simulink model "new_pll_fs"  (Simulink 7.5)
settings: Solver=ode45  StartTime=0.0  StopTime=inf  RelTol=1e-3
undefined symbols (not defined in the file or in its folder): get
libraries: simulink x6, powerlib_extras x2, commsynccomp2 x2, dspsnks4 x2, dsparch4 x1
CloseFcn:
  | rtwprivate ssgencode ModelCloseRequest new_pll_fs
settings Model: Creator=Administrator  LastModifiedBy=kostas777711  SimulationMode=accelerator
settings OptimizationCC: InitFltsAndDblsToZero=on
settings DebuggingCC: SaveWithParameterizedLinksMsg=none  SolverPrmCheckMsg=none  SigSpecEnsureSampleTimeMsg=none  StrictBusMsg=Warning
settings HardwareCC: ProdIntDivRoundTo=Zero  ProdEndianess=LittleEndian  ProdHWDeviceType=32-bit xPC Target (AMD Athlon)  TargetEndianess=LittleEndian  TargetHWDeviceType=MATLAB Host  ProdEqTarget=off
settings RTWCC: SystemTargetFile=accel.tlc  TemplateMakefile=accel_default_tmf  RTWVerbose=off  ProcessScript=accel_make_rtw_hook
settings STFCustomTargetCC: TargetFcnLib=ansi_tfl_tmw.mat  GeneratePreprocessorConditionals=Disable all  SystemTargetFile=accel.tlc

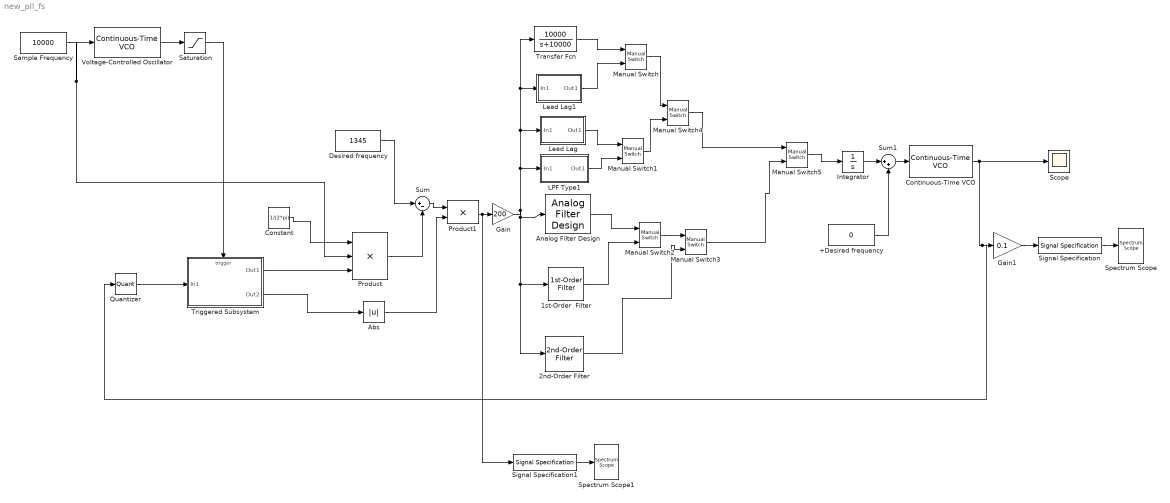
== system new_pll_fs ==
  +Desired frequency : Constant  Value=0  OutDataType=sfix(16)  OutScaling=2^0
  1st-Order  Filter : powerlib_extras/Control  Blocks/1st-Order  Filter  DialogController=POWERSYS.PowerSysDialog  SystemSampleTime=-1  FilterType=Highpass  Tc=12e-3  Initialize=off  Vac_Init=[0.8 -25 60]  Vdc_Init=-0.4  PlotResponse=off  param1=[1 500 1]
  2nd-Order Filter : powerlib_extras/Control  Blocks/2nd-Order Filter  DialogController=POWERSYS.PowerSysDialog  SystemSampleTime=-1  FilterType=Lowpass  Fo=500  Zeta=0.707  Initialize=off  Vac_Init=[1 45 60]  Vdc_Init=-0.5  PlotResponse=off  param1=[1 500 1]
  Abs : Abs  SaturateOnIntegerOverflow=on
  Analog Filter Design : dsparch4/Analog Filter Design  method=Butterworth  filttype=Lowpass  N=4  Wlo=5000  Whi=80  Rp=2  Rs=40
  Constant : Constant  Value=1/(2*pi)  OutDataType=sfix(16)  OutScaling=2^0
  Continuous-Time VCO : commsynccomp2/Continuous-Time VCO  SystemSampleTime=-1  Ac=1  Fc=0  Kc=1  Ph=0
  Desired frequency : Constant  Value=1345  OutDataType=sfix(16)  OutScaling=2^0
  Gain : Gain  Gain=200  ParameterDataType=sfix(16)  ParameterScaling=2^0  OutDataType=sfix(16)  OutScaling=2^0  SaturateOnIntegerOverflow=on  OutDataTypeStr=Inherit: Same as input  ParamDataTypeStr=Inherit: Same as input
  Gain1 : Gain  Gain=0.1  ParameterDataType=sfix(16)  ParameterScaling=2^0  OutDataType=sfix(16)  OutScaling=2^0  SaturateOnIntegerOverflow=on  OutDataTypeStr=Inherit: Same as input  ParamDataTypeStr=Inherit: Same as input
  Integrator : Integrator
  LPF Type1 : Subsystem  TreatAsAtomicUnit=on
  Lead Lag : Subsystem  TreatAsAtomicUnit=on
  Lead Lag1 : Subsystem  TreatAsAtomicUnit=on
  Manual Switch{,2..4} (4 alike) : simulink/Signal Routing/Manual Switch  SystemSampleTime=-1  sw=1  action=0  varsize=off
  Manual Switch1 : simulink/Signal Routing/Manual Switch  SystemSampleTime=-1  sw=0  action=0  varsize=off
  Manual Switch5 : simulink/Signal Routing/Manual Switch  SystemSampleTime=-1  sw=0  action=0  varsize=off
  Product : Product  Inputs=3  OutDataType=sfix(16)  OutScaling=2^0  SaturateOnIntegerOverflow=on  OutDataTypeStr=Inherit: Same as first input
  Product1 : Product  OutDataType=sfix(16)  OutScaling=2^0  SaturateOnIntegerOverflow=on  OutDataTypeStr=Inherit: Same as first input
  Quantizer : Quantizer  QuantizationInterval=2/(2^8)
  Sample Frequency : Constant  Value=10000  OutDataType=sfix(16)  OutScaling=2^0
  Saturation : Saturate  UpperLimit=1  LowerLimit=-1
  Scope : Scope
      settings: TimeRange=0.002973977695167286  YMin=-1  YMax=1
  Signal Specification : SignalSpecification  Dimensions=1  SampleTime=1/10000  OutDataType=sfix(16)  OutScaling=2^0
  Signal Specification1 : SignalSpecification  Dimensions=1  SampleTime=1/10000  OutDataType=sfix(16)  OutScaling=2^0
  Spectrum Scope : dspsnks4/Spectrum Scope  DialogController=dspdialog.SpectrumScope  DialogControllerArgs=DataTag0  SystemSampleTime=-1  ScopeProperties=on  Domain=Frequency  HorizSpan=1  UseBuffer=on  BufferSize=2048  Overlap=64  inpFftLenInherit=on  FFTlength=2048  numAvg=2  DisplayProperties=off  AxisGrid=on  Memory=off  FrameNumber=on  AxisLegend=off  AxisZoom=off  OpenScopeAtSimStart=on  OpenScopeImmediately=off  FigPos=get(0,'defaultfigureposition')  AxisProperties=off  XUnits=Hertz  XRange=[0...Fs/2]  XDisplay=0  InheritXIncr=on  XIncr=1.0  XLabel=Samples  XLimit=Auto  YUnits=dBW/Hertz  XMax=1  XMin=0  YLabel=Magnitude, dB  LineProperties=off  LineColors=[1 0 0]  wintypeSpecScope=Hann  RsSpecScope=50  betaSpecScope=5  winsampSpecScope=Periodic  XAxisParamsVer=6.8
      settings: YMin=-204.6096  YMax=-26.407
  Spectrum Scope1 : dspsnks4/Spectrum Scope  DialogController=dspdialog.SpectrumScope  DialogControllerArgs=DataTag1  SystemSampleTime=-1  ScopeProperties=on  Domain=Frequency  HorizSpan=1  UseBuffer=on  BufferSize=2048  Overlap=64  inpFftLenInherit=on  FFTlength=2048  numAvg=2  DisplayProperties=off  AxisGrid=on  Memory=off  FrameNumber=on  AxisLegend=off  AxisZoom=off  OpenScopeAtSimStart=on  OpenScopeImmediately=off  FigPos=get(0,'defaultfigureposition')  AxisProperties=off  XUnits=Hertz  XRange=[0...Fs/2]  XDisplay=0  InheritXIncr=on  XIncr=1.0  XLabel=Samples  XLimit=Auto  YUnits=dBW/Hertz  XMax=1  XMin=0  YLabel=Magnitude, dB  LineProperties=off  LineStyles=-  LineMarkers=.  wintypeSpecScope=Hann  RsSpecScope=50  betaSpecScope=5  winsampSpecScope=Periodic  XAxisParamsVer=6.8
      settings: YMin=-177.2819  YMax=-38.6723
  Sum : Sum  Inputs=|+-  OutDataType=sfix(16)  OutScaling=2^0  SaturateOnIntegerOverflow=on
  Sum1 : Sum  Inputs=|++  OutDataType=sfix(16)  OutScaling=2^0  SaturateOnIntegerOverflow=on
  Transfer Fcn : TransferFcn  Numerator=[10000]  Denominator=[1 10000]
  Triggered Subsystem : Subsystem  TreatAsAtomicUnit=on
  Voltage-Controlled Oscillator : commsynccomp2/Continuous-Time VCO  SystemSampleTime=-1  Ac=1  Fc=0  Kc=1  Ph=0
  wires:
  Signal Specification/1 -> Spectrum Scope/1
  Gain1/1 -> Signal Specification/1
  Transfer Fcn/1 -> Manual Switch/1
  Lead Lag1/1(Out1) -> Manual Switch/2
  Lead Lag/1(Out1) -> Manual Switch1/1
  LPF Type1/1(Out1) -> Manual Switch1/2
  Analog Filter Design/1 -> Manual Switch2/1
  1st-Order  Filter/1 -> Manual Switch2/2
  Manual Switch2/1 -> Manual Switch3/1
  2nd-Order Filter/1 -> Manual Switch3/2
  Manual Switch/1 -> Manual Switch4/1
  Manual Switch1/1 -> Manual Switch4/2
  Manual Switch4/1 -> Manual Switch5/1
  Continuous-Time VCO/1 -> Scope/1, Gain1/1, Quantizer/1
  Manual Switch3/1 -> Manual Switch5/2
  Signal Specification1/1 -> Spectrum Scope1/1
  Voltage-Controlled Oscillator/1 -> Saturation/1
  Sample Frequency/1 -> Voltage-Controlled Oscillator/1, Product/2
  Desired frequency/1 -> Sum/1
  Product/1 -> Sum/2
  Manual Switch5/1 -> Integrator/1
  Product1/1 -> Gain/1, Signal Specification1/1
  Sum/1 -> Product1/1
  Abs/1 -> Product1/2
  Constant/1 -> Product/1
  Saturation/1 -> Triggered Subsystem/Trigger
  Quantizer/1 -> Triggered Subsystem/1(In1)
  Triggered Subsystem/1(Out1) -> Product/3
  Gain/1 -> Transfer Fcn/1, Lead Lag1/1(In1), Lead Lag/1(In1), LPF Type1/1(In1), Analog Filter Design/1, 1st-Order  Filter/1, 2nd-Order Filter/1
  Triggered Subsystem/2(Out2) -> Abs/1
  Sum1/1 -> Continuous-Time VCO/1
  Integrator/1 -> Sum1/1
  +Desired frequency/1 -> Sum1/2

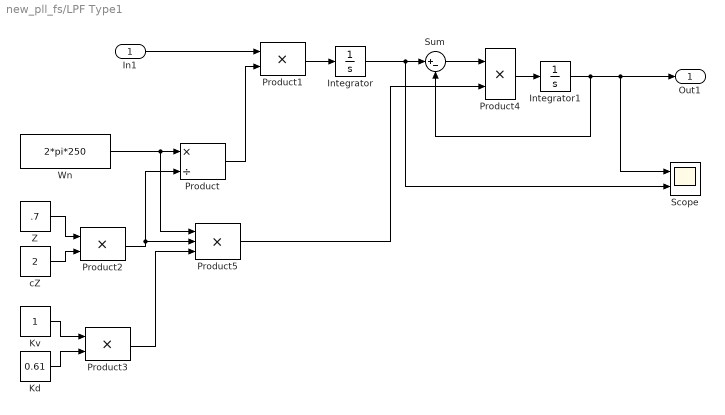
== system new_pll_fs/LPF Type1 ==
  In1 : Inport  OutDataType=sfix(16)  OutScaling=2^0
  Integrator : Integrator  InitialCondition=2500  LimitOutput=on  UpperSaturationLimit=5000  LowerSaturationLimit=10
  Integrator1 : Integrator  InitialCondition=100  LimitOutput=on  UpperSaturationLimit=5000  LowerSaturationLimit=10
  Kd : Constant  Value=0.61  OutDataType=sfix(16)  OutScaling=2^0
  Kv : Constant  OutDataType=sfix(16)  OutScaling=2^0
  Product : Product  Inputs=*/  OutDataType=sfix(16)  OutScaling=2^0  RndMeth=Nearest  SaturateOnIntegerOverflow=on  OutDataTypeStr=Inherit: Same as first input
  Product1 : Product  OutDataType=sfix(16)  OutScaling=2^0  SaturateOnIntegerOverflow=on  OutDataTypeStr=Inherit: Same as first input
  Product2 : Product  OutDataType=sfix(16)  OutScaling=2^0  SaturateOnIntegerOverflow=on  OutDataTypeStr=Inherit: Same as first input
  Product3 : Product  OutDataType=sfix(16)  OutScaling=2^0  SaturateOnIntegerOverflow=on  OutDataTypeStr=Inherit: Same as first input
  Product4 : Product  Inputs=**  OutDataType=sfix(16)  OutScaling=2^0  SaturateOnIntegerOverflow=on  OutDataTypeStr=Inherit: Same as first input
  Product5 : Product  Inputs=***  OutDataType=sfix(16)  OutScaling=2^0  RndMeth=Nearest  SaturateOnIntegerOverflow=on  OutDataTypeStr=Inherit: Same as first input
  Scope : Scope  NumInputPorts=2
      settings: TimeRange=0.01  YMin=748.5~748  YMax=751~753  SaveName=ScopeData2
  Sum : Sum  Inputs=|+-  OutDataType=sfix(16)  OutScaling=2^0  SaturateOnIntegerOverflow=on
  Wn : Constant  Value=2*pi*250  OutDataType=sfix(16)  OutScaling=2^0
  Z : Constant  Value=.7  OutDataType=sfix(16)  OutScaling=2^0
  cZ : Constant  Value=2  OutDataType=sfix(16)  OutScaling=2^0
  Out1 : Outport  OutDataType=sfix(16)  OutScaling=2^0
  wires:
  Product/1 -> Product1/2
  Z/1 -> Product2/1
  cZ/1 -> Product2/2
  Kv/1 -> Product3/1
  Kd/1 -> Product3/2
  Wn/1 -> Product/1, Product5/1
  Product1/1 -> Integrator/1
  Integrator/1 -> Sum/1, Scope/2
  In1/1 -> Product1/1
  Integrator1/1 -> Sum/2, Out1/1, Scope/1
  Sum/1 -> Product4/1
  Product4/1 -> Integrator1/1
  Product2/1 -> Product/2, Product5/2
  Product3/1 -> Product5/3
  Product5/1 -> Product4/2

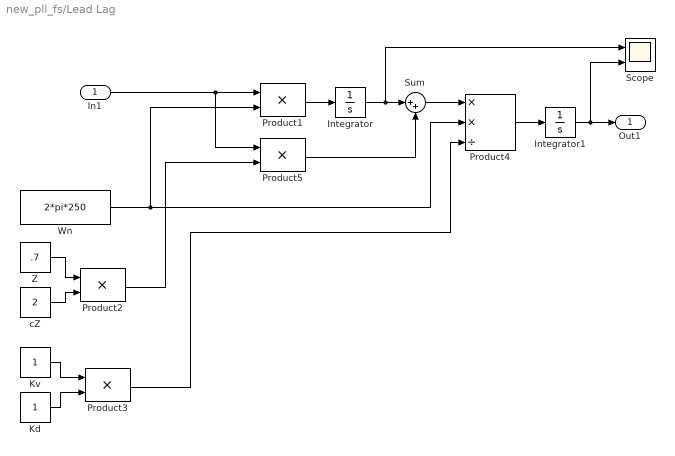
== system new_pll_fs/Lead Lag ==
  In1 : Inport  OutDataType=sfix(16)  OutScaling=2^0
  Integrator : Integrator  UpperSaturationLimit=10  LowerSaturationLimit=-10  ZeroCross=off
  Integrator1 : Integrator  InitialCondition=1000  LimitOutput=on  UpperSaturationLimit=5000  LowerSaturationLimit=10
  Kd : Constant  OutDataType=sfix(16)  OutScaling=2^0
  Kv : Constant  OutDataType=sfix(16)  OutScaling=2^0
  Product{1..3,5} (4 alike) : Product  OutDataType=sfix(16)  OutScaling=2^0  SaturateOnIntegerOverflow=on  OutDataTypeStr=Inherit: Same as first input
  Product4 : Product  Inputs=**/  OutDataType=sfix(16)  OutScaling=2^0  SaturateOnIntegerOverflow=on  OutDataTypeStr=Inherit: Same as first input
  Scope : Scope  NumInputPorts=2
      settings: TimeRange=0.02  YMin=-10~490  YMax=7.5~515  SaveName=ScopeData3
  Sum : Sum  Inputs=|++  OutDataType=sfix(16)  OutScaling=2^0  SaturateOnIntegerOverflow=on
  Wn : Constant  Value=2*pi*250  OutDataType=sfix(16)  OutScaling=2^0
  Z : Constant  Value=.7  OutDataType=sfix(16)  OutScaling=2^0
  cZ : Constant  Value=2  OutDataType=sfix(16)  OutScaling=2^0
  Out1 : Outport  OutDataType=sfix(16)  OutScaling=2^0
  wires:
  Z/1 -> Product2/1
  cZ/1 -> Product2/2
  Kv/1 -> Product3/1
  Kd/1 -> Product3/2
  Wn/1 -> Product1/2, Product4/2
  Product1/1 -> Integrator/1
  In1/1 -> Product1/1, Product5/1
  Integrator/1 -> Sum/1, Scope/1
  Product2/1 -> Product5/2
  Product5/1 -> Sum/2
  Sum/1 -> Product4/1
  Product3/1 -> Product4/3
  Product4/1 -> Integrator1/1
  Integrator1/1 -> Out1/1, Scope/2

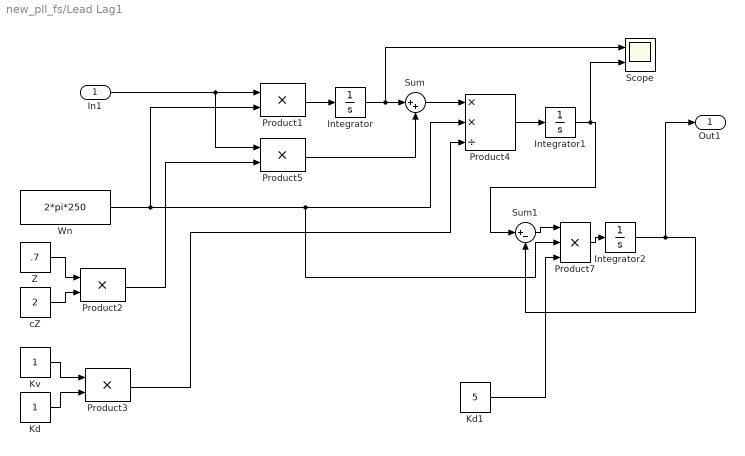
== system new_pll_fs/Lead Lag1 ==
  In1 : Inport  OutDataType=sfix(16)  OutScaling=2^0
  Integrator : Integrator  UpperSaturationLimit=10  LowerSaturationLimit=-10  ZeroCross=off
  Integrator1 : Integrator  InitialCondition=1000  LimitOutput=on  UpperSaturationLimit=5000  LowerSaturationLimit=10
  Integrator2 : Integrator  UpperSaturationLimit=10  LowerSaturationLimit=-10  ZeroCross=off
  Kd : Constant  OutDataType=sfix(16)  OutScaling=2^0
  Kd1 : Constant  Value=5  OutDataType=sfix(16)  OutScaling=2^0
  Kv : Constant  OutDataType=sfix(16)  OutScaling=2^0
  Product{1..3,5} (4 alike) : Product  OutDataType=sfix(16)  OutScaling=2^0  SaturateOnIntegerOverflow=on  OutDataTypeStr=Inherit: Same as first input
  Product4 : Product  Inputs=**/  OutDataType=sfix(16)  OutScaling=2^0  SaturateOnIntegerOverflow=on  OutDataTypeStr=Inherit: Same as first input
  Product7 : Product  Inputs=***  OutDataType=sfix(16)  OutScaling=2^0  SaturateOnIntegerOverflow=on  OutDataTypeStr=Inherit: Same as first input
  Scope : Scope  NumInputPorts=2
      settings: TimeRange=0.02  YMin=-126.35~10  YMax=-126.175~10  SaveName=ScopeData3
  Sum : Sum  Inputs=|++  OutDataType=sfix(16)  OutScaling=2^0  SaturateOnIntegerOverflow=on
  Sum1 : Sum  Inputs=|+-  OutDataType=sfix(16)  OutScaling=2^0  SaturateOnIntegerOverflow=on
  Wn : Constant  Value=2*pi*250  OutDataType=sfix(16)  OutScaling=2^0
  Z : Constant  Value=.7  OutDataType=sfix(16)  OutScaling=2^0
  cZ : Constant  Value=2  OutDataType=sfix(16)  OutScaling=2^0
  Out1 : Outport  OutDataType=sfix(16)  OutScaling=2^0
  wires:
  Integrator1/1 -> Scope/2, Sum1/1
  Product4/1 -> Integrator1/1
  Product3/1 -> Product4/3
  Sum/1 -> Product4/1
  Product5/1 -> Sum/2
  Product2/1 -> Product5/2
  Integrator/1 -> Scope/1, Sum/1
  In1/1 -> Product5/1, Product1/1
  Product1/1 -> Integrator/1
  Wn/1 -> Product1/2, Product4/2, Product7/2
  Kd/1 -> Product3/2
  Kv/1 -> Product3/1
  cZ/1 -> Product2/2
  Z/1 -> Product2/1
  Integrator2/1 -> Out1/1, Sum1/2
  Sum1/1 -> Product7/1
  Product7/1 -> Integrator2/1
  Kd1/1 -> Product7/3

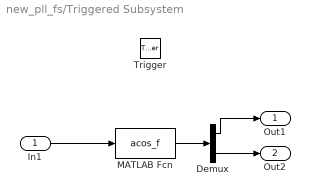
== system new_pll_fs/Triggered Subsystem ==
  In1 : Inport  OutDataType=sfix(16)  OutScaling=2^0
  Trigger : TriggerPort
  Demux : Demux  Outputs=2
  MATLAB Fcn : MATLABFcn  MATLABFcn=acos_f
  Out1 : Outport  OutDataType=sfix(16)  OutScaling=2^0
  Out2 : Outport  Port=2  OutDataType=sfix(16)  OutScaling=2^0
  wires:
  In1/1 -> MATLAB Fcn/1
  MATLAB Fcn/1 -> Demux/1
  Demux/1 -> Out1/1
  Demux/2 -> Out2/1
